simulink model "car_model_FIXED"  (R2022b)
settings: Solver=VariableStepAuto  StartTime=0.0  StopTime=60  RelTol=1e-3
values from neighbouring files (symbols this model uses):
  ABS_MAX_TORQUE = [25 25 25 25]    [Startup.m]
  ABS_MAX_TRQ_CMD = dot(ABS_MAX_TORQUE, MOTOR_ENABLE)    [Startup.m]
  ABS_MIN_TORQUE = [0.01 0.01 0.01 0.01]    [Startup.m]
  acc_IC = 0    [Startup.m]
  ACCELERATION_MAX = 30    [Startup.m]
  ang_IC = 0    [Startup.m]
  ang_vel_IC = 0    [Startup.m]
  ax = Reference_Signals.Chassis_Acceleration_VNED.ax.Data(:)    [Simulation_Data_Parse.m]    (also in Vehicle_Sim_Parse.m)
  ay = Reference_Signals.Chassis_Acceleration_VNED.ay.Data(:)    [Simulation_Data_Parse.m]    (also in Vehicle_Sim_Parse.m)
  az = Reference_Signals.Chassis_Acceleration_VNED.az.Data(:)    [Simulation_Data_Parse.m]    (also in Vehicle_Sim_Parse.m)
  battery_current_IC = 0    [Startup.m]
  BATTERY_CURRENT_MAX = 140    [Startup.m]
  BATTERY_CURRENT_MIN = 0    [Startup.m]
  battery_FT_IC = 300    [Startup.m]
  battery_T_IC = 300    [Startup.m]
  BATTERY_TEMPERATURE_MAX = 60    [Startup.m]
  BATTERY_TEMPERATURE_MIN = 0    [Startup.m]
  battery_voltage_IC = Ns*max(Em)    [Startup.m]
  BATTERY_VOLTAGE_MAX = 340    [Startup.m]
  BATTERY_VOLTAGE_MIN = 60    [Startup.m]
  Brake_Pressure_IC = 1    [Startup.m]
  ccl_IC = 0    [Startup.m]
  CENTER_STEER_ANGLE_MAX = 130    [Startup.m]
  covarience_matrix_IC = Simulink.Parameter(eye(28)./1000)    [Startup.m]
  dcl_IC = 140    [Startup.m]
  DCL_MAX = 130    [Startup.m]
  DCL_MIN = 0    [Startup.m]
  driver_t = 0.015    [Startup.m]
  fusion_t = Simulink.Parameter(0.01)    [Startup.m]
  fusion_t_sim = fusion_t.copy    [Startup.m]
  Fz_IC = m_all*g/4    [Startup.m]
  g = 9.81    [Startup.m]
  gps_hz = 0.01    [Startup.m]
  gps_ratio = Simulink.Parameter(gps_hz / imu_hz.Value)    [Startup.m]
  imu_hz = fusion_t.copy    [Startup.m]
  location_lla_IC = Simulink.Parameter([40.437675, -86.943750, 200])    [Startup.m]
  MAG_MAX = 200    [Startup.m]
  Max_Brake_Pressure = 10^8    (= 100000000)    [Startup.m]
  Max_Driver_Input = 1    [Startup.m]
  MAX_DTHETA_DRIVER = 360    [Startup.m]
  MAX_STEERING_ADJUST = 15    [Startup.m]
  Min_Brake_Pressure = 1    [Startup.m]
  Min_Driver_Input = 0    [Startup.m]
  motor_current_IC = 0    [Startup.m]
  MOTOR_CURRENT_MAX = 70    [Startup.m]
  MOTOR_CURRENT_MIN = 0    [Startup.m]
  MOTOR_ENABLE = [0 0 1 1]    [Startup.m]
  motor_FT_IC = 300    [Startup.m]
  motor_T_IC = 300    [Startup.m]
  MOTOR_TEMPERATURE_MAX = 100    [Startup.m]
  MOTOR_TEMPERATURE_MIN = 0    [Startup.m]
  motor_voltage_IC = 332    [Startup.m]
  MOTOR_VOLTAGE_MAX = 340    [Startup.m]
  MOTOR_VOLTAGE_MIN = 90    [Startup.m]
  omega_IC = 0    [Startup.m]
  OMEGA_MAX = 150    [Startup.m]
  OMEGA_MIN = 0    [Startup.m]
  ORIENTATION_MAX = 360    [Startup.m]
  pos_IC = 0    [Startup.m]
  POS_MAX = 300    [Startup.m]
  rho = 1.225    [Startup.m]
  selected_maxvm = MIN_TRACK_DATA.(event_names(10))    [Startup.m]
  selected_sweep = ALL_SWEEP_DATA.(sweep_names(1))    [Startup.m]
  selected_track = ALL_TRACK_DATA.(event_names(10))    [Startup.m]
  shock_length_IC = 0.1    [Startup.m]
  SHOCK_LENGTH_MAX = 0.25    [Startup.m]
  SHOCK_LENGTH_MIN = 0    [Startup.m]
  state_IC = zeros(28,1)    [Startup.m]
  theta_IC = 0    [Startup.m]
  TRACTION_ENABLE = 0    [Startup.m]
  TVS_ENABLE = 0    [Startup.m]
  tvs_t = 0.015    [Startup.m]
  tvs_t_sim = tvs_t    (= 0.015)    [Startup.m]
  Tx_I = 0    [Startup.m]
  vel_IC = [0 0 0]    [Startup.m]
  VELOCITY_MAX = 30    [Startup.m]
  X = Reference_Signals.Chassis_Position.X.Data(:)    [Simulation_Data_Parse.m]    (also in Vehicle_Sim_Parse.m = Chassis_Signals.InertFrm.Cg.Disp.X.Data(:))
  Y = Reference_Signals.Chassis_Position.Y.Data(:)    [Simulation_Data_Parse.m]    (also in Vehicle_Sim_Parse.m = Chassis_Signals.InertFrm.Cg.Disp.Y.Data(:))
  YAW_ENABLE = 1    [Startup.m]
  YAW_MAX = 2.5    [Startup.m]
undefined symbols (not defined in the file or in its folder): ActSuspDutyCycle, Aeq_left, Aeq_right, alpha_error, ang_acc_hystersesis, area_air, axb, br, brake_bias, covA, covG, covM, covP, covV, CURRENT_BUFFER, cy_sweep, dB, deadband_angle, dIndex, DiscIntNeverNeededParam, dt_OFF, dt_ON, dTx, dx, dZ, efficiency_grid, F0z, forward_look_straight, forward_look_turn, Fz_sweep, GAIN_ABS, gearbox_efficiency, gr, I, I_Driver, IMU_accel, IMU_gyro, IMU_mag, IMUNED2VNED, indicies, IYY, kx_sweep, l, lambda_star, low_V_SA, lr, m_all, m_body, m_unsprung, MAGNED2VNED, MAX_I_Driver, max_yaw, min_velocity_regen, motorControllerCurve, motorTempCurve, motorTempX, mu_star, mx_sweep, my_sweep, noise_state ... (+40)
libraries: fl_lib x82, nesl_utility x32, vehdynlibtire x10, vehdynlibsuspension x8, simulink x5, autolibutils x5, sharedtransform x5, sdl_lib x4, EngineCoolingComponents_lib x4, slpidlib x3, SimscapeFluids_lib x3, shared6dof x2
(part 8 of 14)

== system car_model_FIXED/Control Systems/TVS/Yaw Controller/Integrator ==
  yaw_error : Inport
  windup : Inport  Port=2
  P_control : Inport  Port=3
  control_signal : Inport  Port=4
  Constant2 : Constant  Value=0
  Gain : Gain  Gain=I*tvs_t
  Gain1 : Gain  Gain=0.5
  Sum1 : Sum  Inputs=|+-
  Sum2 : Sum  Inputs=|++
  Sum3 : Sum  Inputs=|++
  Switch1 : Switch  Criteria=u2 > Threshold  SaturateOnIntegerOverflow=off  InputSameDT=off
  Switch2 : Switch  Criteria=u2 > Threshold  SaturateOnIntegerOverflow=off  InputSameDT=off
  Unit Delay1 : UnitDelay  SampleTime=-1  HasFrameUpgradeWarning=on
  Unit Delay2 : UnitDelay  SampleTime=-1  HasFrameUpgradeWarning=on
  I_control : Outport
  wires:
  Constant2/1 -> Switch1/1
  windup/1 -> Switch1/2, Switch2/2
  Gain/1 -> Unit Delay1/1, Sum3/1
  Switch1/1 -> Sum2/1
  Gain1/1 -> Switch1/3
  Sum2/1 -> Switch2/3, I_control/1
  Unit Delay1/1 -> Sum3/2
  Sum3/1 -> Gain1/1
  yaw_error/1 -> Gain/1
  control_signal/1 -> Sum1/1
  P_control/1 -> Sum1/2
  Sum1/1 -> Switch2/1
  Switch2/1 -> Unit Delay2/1
  Unit Delay2/1 -> Sum2/2

== system car_model_FIXED/Control Systems/TVS/Yaw Controller/Windup Hysteresis ==
  max_ang_acc : Inport
  min_ang_acc : Inport  Port=2
  control_signal : Inport  Port=3
  AND : Logic  IconShape=distinctive  AllPortsSameDT=off  OutDataTypeStr=boolean
  Bias : Bias  Bias=-ang_acc_hystersesis  SaturateOnIntegerOverflow=off
  Bias1 : Bias  Bias=ang_acc_hystersesis  SaturateOnIntegerOverflow=off
  Bias2 : Bias  Bias=ang_acc_hystersesis  SaturateOnIntegerOverflow=off
  Bias3 : Bias  Bias=-ang_acc_hystersesis  SaturateOnIntegerOverflow=off
  Less Than : RelationalOperator  Operator=>  OutDataTypeStr=boolean  RndMeth=Simplest  InputSameDT=off
  Less Than1 : RelationalOperator  Operator=<  OutDataTypeStr=boolean  RndMeth=Simplest  InputSameDT=off
  Less Than2 : RelationalOperator  Operator=<  OutDataTypeStr=boolean  RndMeth=Simplest  InputSameDT=off
  Less Than3 : RelationalOperator  Operator=>  OutDataTypeStr=boolean  RndMeth=Simplest  InputSameDT=off
  NOT : Logic  Operator=NOT  IconShape=distinctive  AllPortsSameDT=off  OutDataTypeStr=boolean
  OR : Logic  Operator=OR  IconShape=distinctive  AllPortsSameDT=off  OutDataTypeStr=boolean
  Switch : Switch  Criteria=u2 > Threshold  SaturateOnIntegerOverflow=off  InputSameDT=off
  Switch1 : Switch  Criteria=u2 > Threshold  SaturateOnIntegerOverflow=off  InputSameDT=off
  Unit Delay : UnitDelay  SampleTime=-1  HasFrameUpgradeWarning=on
  windup : Outport
  wires:
  min_ang_acc/1 -> Bias1/1, Bias3/1
  max_ang_acc/1 -> Bias/1, Bias2/1
  Less Than/1 -> AND/1
  Less Than1/1 -> AND/2
  Bias/1 -> Less Than1/2
  Bias1/1 -> Less Than/2
  AND/1 -> Switch/2, NOT/1
  Unit Delay/1 -> Switch/3, windup/1  "windup"
  Bias3/1 -> Less Than2/2
  Bias2/1 -> Less Than3/2
  OR/1 -> Switch1/2, Switch1/1
  Less Than3/1 -> OR/2
  Less Than2/1 -> OR/1
  control_signal/1 -> Less Than2/1, Less Than3/1, Less Than1/1, Less Than/1
  NOT/1 -> Switch/1
  Switch/1 -> Switch1/3
  Switch1/1 -> Unit Delay/1  "windup"

== system car_model_FIXED/Driver & Environment/Longitudinal Control/ABS/ABS system ==
  lambda0 : Inport
  Vx : Inport  Port=2
  omega : Inport  Port=3
  ABS_ENABLE : Inport  Port=4
  Bias : Bias  Bias=1  SaturateOnIntegerOverflow=off
  Constant : Constant  Value=0
  Constant1 : Constant  Value=mu_star
  Divide : Product  Inputs=*/
  Equal : RelationalOperator  Operator===  OutDataTypeStr=boolean  RndMeth=Simplest  InputSameDT=off
  Gain : Gain  Gain=-1
  Gain1 : Gain  Gain=eps
  Gain2 : Gain  Gain=-g
  Gain8 : Gain  Gain=RE
  MATLAB Function : MATLAB Function  TreatAsAtomicUnit=on  SystemSampleTime=driver_t
  MATLAB Function1 : MATLAB Function  TreatAsAtomicUnit=on
  Product : Product  Inputs=1
  Product1 : Product
  Product2 : Product
  Reshape : Reshape  OutputDimensionality=Row vector (2-D)
  Reshape1 : Reshape  OutputDimensionality=Row vector (2-D)
  Sum : Sum  Inputs=|++
  Switch : Switch  Criteria=u2 ~= 0  SaturateOnIntegerOverflow=off  InputSameDT=off
  Transpose : Math  Operator=transpose
  mu : Outport
  Bx : Outport  Port=2
  OFF_FLAG : Outport  Port=3
  wires:
  omega/1 -> Reshape1/1, Product1/2  "w"
  Product2/1 -> Sum/1, Equal/1, MATLAB Function/3(v)
  MATLAB Function/1(tau) -> Bx/1  "braking torque"
  Bias/1 -> MATLAB Function/6(lambda), MATLAB Function1/1(u)  "lambda"
  Gain8/1 -> Divide/1
  lambda0/1 -> Transpose/1
  Divide/1 -> Gain/1
  Sum/1 -> Divide/2
  Equal/1 -> Gain1/1
  Constant/1 -> Equal/2
  Gain/1 -> Bias/1
  Gain1/1 -> Sum/2
  Transpose/1 -> MATLAB Function/4(lambda0)
  Reshape/1 -> MATLAB Function/1(w_fake), Gain8/1
  MATLAB Function1/1(y) -> Product/1  "mu"
  Gain2/1 -> MATLAB Function/5(vdot)
  MATLAB Function/2(d) -> OFF_FLAG/1
  Product/1 -> Switch/1, Gain2/1
  Product1/1 -> Reshape/1
  Switch/1 -> mu/1
  Constant1/1 -> Switch/3
  Vx/1 -> Product2/2
  ABS_ENABLE/1 -> Switch/2, Product2/1, Product1/1
  Reshape1/1 -> MATLAB Function/2(w)

== system car_model_FIXED/Vehicle Model/Powertrain/Motor Cooling Loop/Air Stream ==
  V : Inport
  fan command : Inport  Port=2
  Air density [kg/m^3] : Constant  Value=rho
  Constant : Constant
  Product : Product  Inputs=3
  Radiator area [m^2] : Constant  Value=area_air
  Simulink-PS Converter1 : nesl_utility/Simulink-PS Converter  PhysicalDomain=network_engine_domain  SubClassName=ps_input  LeftPortType=input  RightPortType=output  PseudoPeriodic=off  Frequencies=[]  NoiseDistribution=none  NoiseParameters=[]  Unit=kg/s  AffineConversion=off  FilteringAndDerivatives=filter  SimscapeFilterOrder=1  InputFilterTimeConstant=0.01  UdotUserProvided=0
  Sum : Sum  Inputs=|++
  Terminator : Terminator
  mdot : PMIOPort  Side=Right
  wires:
  Constant/1 -> Sum/1
  Product/1 -> Simulink-PS Converter1/1
  Radiator area [m^2]/1 -> Product/2
  Air density [kg/m^3]/1 -> Product/3
  Sum/1 -> Product/1
  fan command/1 -> Sum/2
  V/1 -> Terminator/1
  connections:
  mdot/RConn1 -- Simulink-PS Converter1/RConn1

== system car_model_FIXED/Vehicle Model/Powertrain/Motor Cooling Loop/Expansion Tank ==
  Expansion Tank : fl_lib/Thermal Liquid/Elements/Translational Mechanical Converter (TL)  mech_orientation=1  displacement_spec=foundation.enum.DisplacementSpec.Calculate  x0=0 m  interface_area=pi*0.01^2 m^2  dead_volume=pi*0.01^2 * 0.001 m^3  environment_spec=foundation.enum.pressure_spec.specified  environment_pressure=1 atm  dynamic_compressibility=0  p0=1 atm  T0=300 K
      settings: InternalSimscapePortConfiguration="{\"Bottom\":[],\"Left\":[{\"id\":\"A\",\"label\":\"A\",\"type\":\"foundation.thermal_liquid.thermal_liquid\"},{\"id\":\"C\",\"label\":\"C\",\"type\":\"foundation.mechanical.translational.translational\"},{\"id\":\"H\",\"label\":\"H\",\"type\":\"foundation.thermal.thermal\"}],\"Right\":[{\"id\":\"R\",\"label\":\"R\",\"type\":\"foundation.mechanical.translational.translational\"}],\"Top\":[]}"
  Ideal Force Source : fl_lib/Mechanical/Mechanical Sources/Ideal Force Source
  Mechanical Translational Reference : fl_lib/Mechanical/Translational Elements/Mechanical Translational Reference
  Mechanical Translational Reference1 : fl_lib/Mechanical/Translational Elements/Mechanical Translational Reference
  PS Gain : fl_lib/Physical Signals/Functions/PS Gain  gain=-1
  PS Product : fl_lib/Physical Signals/Functions/PS Product
  Perfect Insulator : fl_lib/Thermal/Thermal Elements/Perfect Insulator  T_specify=off  T_priority=None  T=0 K  T_nominal_specify=off  T_nominal_unit=K  T_nominal_value=1
  Relief Pressure (Absolute) : fl_lib/Physical Signals/Sources/PS Constant  constant=2e5
  Relief Valve : fl_lib/Thermal Liquid/Elements/Local Restriction (TL)  restriction_type=foundation.enum.restriction_type.fixed  restriction_area=pi*0.005^2 m^2  min_area=1e-10 m^2  max_area=0.005 m^2  area=pi*0.01^2 m^2  Cd=0.7  pressure_recovery=simscape.enum.onoff.on  Re_c=12
  Tank Area : fl_lib/Physical Signals/Sources/PS Constant  constant=pi*0.01^2
  Translational Hard Stop : fl_lib/Mechanical/Translational Elements/Translational Hard Stop  upper_bnd=100 m  lower_bnd=0 m  stiff_up=1e6 N/m  stiff_low=1e6 N/m  D_up=0 N/(m/s)  D_low=0 N/(m/s)  model=3  transition=0.1 mm  v_specify=off  v_priority=None  v=0 m/s  v_nominal_specify=off  v_nominal_unit=m/s  v_nominal_value=1  f_specify=off  f_priority=None  f=0 N  f_nominal_specify=off  f_nominal_unit=N  f_nominal_value=1  x_specify=on  x_priority=High  x=0 m  x_nominal_specify=off  x_nominal_unit=m  x_nominal_value=1
  P : PMIOPort  Side=Left
  connections:
  Mechanical Translational Reference/LConn1 -- Expansion Tank/LConn2
  Perfect Insulator/LConn1 -- Expansion Tank/LConn3
  Relief Valve/LConn1 -- P/RConn1
  Relief Valve/RConn1 -- Expansion Tank/LConn1
  Ideal Force Source/LConn1 -- Expansion Tank/RConn1 -- Translational Hard Stop/LConn1
  Mechanical Translational Reference1/LConn1 -- Translational Hard Stop/RConn1 -- Ideal Force Source/RConn2
  PS Gain/LConn1 -- PS Product/RConn1
  PS Gain/RConn1 -- Ideal Force Source/RConn1
  PS Product/LConn1 -- Tank Area/RConn1
  Relief Pressure (Absolute)/RConn1 -- PS Product/LConn2

== system car_model_FIXED/Vehicle Model/Powertrain/Motor Cooling Loop/Expansion Tank1 ==
  Expansion Tank : fl_lib/Thermal Liquid/Elements/Translational Mechanical Converter (TL)  mech_orientation=1  displacement_spec=foundation.enum.DisplacementSpec.Calculate  x0=0 m  interface_area=pi*0.01^2 m^2  dead_volume=pi*0.01^2 * 0.001 m^3  environment_spec=2  environment_pressure=1 atm  dynamic_compressibility=0  p0=1 atm  T0=300 K
      settings: InternalSimscapePortConfiguration="{\"Bottom\":[],\"Left\":[{\"id\":\"A\",\"label\":\"A\",\"type\":\"foundation.thermal_liquid.thermal_liquid\"},{\"id\":\"C\",\"label\":\"C\",\"type\":\"foundation.mechanical.translational.translational\"},{\"id\":\"H\",\"label\":\"H\",\"type\":\"foundation.thermal.thermal\"}],\"Right\":[{\"id\":\"R\",\"label\":\"R\",\"type\":\"foundation.mechanical.translational.translational\"}],\"Top\":[]}"
  Ideal Force Source : fl_lib/Mechanical/Mechanical Sources/Ideal Force Source
  Mechanical Translational Reference : fl_lib/Mechanical/Translational Elements/Mechanical Translational Reference
  Mechanical Translational Reference1 : fl_lib/Mechanical/Translational Elements/Mechanical Translational Reference
  PS Gain : fl_lib/Physical Signals/Functions/PS Gain  gain=-1
  PS Product : fl_lib/Physical Signals/Functions/PS Product
  Perfect Insulator : fl_lib/Thermal/Thermal Elements/Perfect Insulator  T_specify=off  T_priority=None  T=0 K  T_nominal_specify=off  T_nominal_unit=K  T_nominal_value=1
  Relief Pressure (Absolute) : fl_lib/Physical Signals/Sources/PS Constant  constant=2e5
  Relief Valve : fl_lib/Thermal Liquid/Elements/Local Restriction (TL)  restriction_type=foundation.enum.restriction_type.fixed  restriction_area=pi*0.005^2 m^2  min_area=1e-10 m^2  max_area=0.005 m^2  area=pi*0.01^2 m^2  Cd=0.7  pressure_recovery=simscape.enum.onoff.on  Re_c=12
  Tank Area : fl_lib/Physical Signals/Sources/PS Constant  constant=pi*0.01^2
  Translational Hard Stop : fl_lib/Mechanical/Translational Elements/Translational Hard Stop  upper_bnd=100 m  lower_bnd=0 m  stiff_up=1e6 N/m  stiff_low=1e6 N/m  D_up=0 N/(m/s)  D_low=0 N/(m/s)  model=3  transition=0.1 mm  v_specify=off  v_priority=None  v=0 m/s  v_nominal_specify=off  v_nominal_unit=m/s  v_nominal_value=1  f_specify=off  f_priority=None  f=0 N  f_nominal_specify=off  f_nominal_unit=N  f_nominal_value=1  x_specify=on  x_priority=High  x=0 m  x_nominal_specify=off  x_nominal_unit=m  x_nominal_value=1
  P : PMIOPort  Side=Left
  connections:
  Mechanical Translational Reference/LConn1 -- Expansion Tank/LConn2
  Perfect Insulator/LConn1 -- Expansion Tank/LConn3
  Relief Valve/LConn1 -- P/RConn1
  Relief Valve/RConn1 -- Expansion Tank/LConn1
  Ideal Force Source/LConn1 -- Expansion Tank/RConn1 -- Translational Hard Stop/LConn1
  Mechanical Translational Reference1/LConn1 -- Translational Hard Stop/RConn1 -- Ideal Force Source/RConn2
  PS Gain/LConn1 -- PS Product/RConn1
  PS Gain/RConn1 -- Ideal Force Source/RConn1
  PS Product/LConn1 -- Tank Area/RConn1
  Relief Pressure (Absolute)/RConn1 -- PS Product/LConn2

== system car_model_FIXED/Vehicle Model/Powertrain/Motor Cooling Loop/Motor FL ==
  Fluid Jacket : EngineCoolingComponents_lib/Fluid Jacket  volume=5.2e-6 m^3  length=0.087 m  area=pi*(0.012/2)^2 m^2  loss_coefficient=1  heat_transfer_area=22925 mm^2  Nu_coeff=[0.3, 0.8, 0.33]  p_I_specify=off  p_I_priority=High  p_I=1 atm  p_I_nominal_specify=off  p_I_nominal_unit=MPa  p_I_nominal_value=1  T_I_specify=on  T_I_priority=High  T_I=300 K  T_I_nominal_specify=off  T_I_nominal_unit=K  T_I_nominal_value=1
      settings: InternalSimscapePortConfiguration="{\"Bottom\":[],\"Left\":[{\"id\":\"A\",\"label\":\"A\",\"type\":\"foundation.thermal_liquid.thermal_liquid\"},{\"id\":\"H\",\"label\":\"H\",\"type\":\"foundation.thermal.thermal\"}],\"Right\":[{\"id\":\"B\",\"label\":\"B\",\"type\":\"foundation.thermal_liquid.thermal_liquid\"}],\"Top\":[]}"
  Piston Thermal Mass : fl_lib/Thermal/Thermal Elements/Thermal Mass  mass=3.1 kg  sp_heat=184.91 J/kg/K  num_ports=foundation.enum.numPorts2.one  T_specify=on  T_priority=High  T=300 K  T_nominal_specify=off  T_nominal_unit=K  T_nominal_value=1  Q_specify=off  Q_priority=None  Q=0 W  Q_nominal_specify=off  Q_nominal_unit=W  Q_nominal_value=1
  Sensor : Subsystem
      mask Display: disp('T');
  Heat In : PMIOPort  Side=Left
  Fluid In : PMIOPort  Port=2  Side=Left
  Fluid Out : PMIOPort  Port=3  Side=Right
  connections:
  Fluid Jacket/RConn1 -- Fluid Out/RConn1
  Fluid Jacket/LConn1 -- Fluid In/RConn1
  Fluid Jacket/LConn2 -- Sensor/LConn1 -- Heat In/RConn1 -- Piston Thermal Mass/LConn1

== system car_model_FIXED/Vehicle Model/Powertrain/Motor Cooling Loop/Motor FR ==
  Fluid Jacket : EngineCoolingComponents_lib/Fluid Jacket  volume=5.2e-6 m^3  length=0.087 m  area=pi*(0.012/2)^2 m^2  loss_coefficient=1  heat_transfer_area=22925 mm^2  Nu_coeff=[0.3, 0.8, 0.33]  p_I_specify=off  p_I_priority=High  p_I=1 atm  p_I_nominal_specify=off  p_I_nominal_unit=MPa  p_I_nominal_value=1  T_I_specify=on  T_I_priority=High  T_I=300 K  T_I_nominal_specify=off  T_I_nominal_unit=K  T_I_nominal_value=1
      settings: InternalSimscapePortConfiguration="{\"Bottom\":[],\"Left\":[{\"id\":\"A\",\"label\":\"A\",\"type\":\"foundation.thermal_liquid.thermal_liquid\"},{\"id\":\"H\",\"label\":\"H\",\"type\":\"foundation.thermal.thermal\"}],\"Right\":[{\"id\":\"B\",\"label\":\"B\",\"type\":\"foundation.thermal_liquid.thermal_liquid\"}],\"Top\":[]}"
  Piston Thermal Mass : fl_lib/Thermal/Thermal Elements/Thermal Mass  mass=3.1 kg  sp_heat=184.91 J/kg/K  num_ports=foundation.enum.numPorts2.one  T_specify=on  T_priority=High  T=300 K  T_nominal_specify=off  T_nominal_unit=K  T_nominal_value=1  Q_specify=off  Q_priority=None  Q=0 W  Q_nominal_specify=off  Q_nominal_unit=W  Q_nominal_value=1
  Sensor : Subsystem
      mask Display: disp('T');
  Fluid Out : PMIOPort  Side=Left
  Heat In : PMIOPort  Port=2  Side=Left
  Fluid In : PMIOPort  Port=3  Side=Right
  connections:
  Fluid Jacket/RConn1 -- Fluid Out/RConn1
  Fluid Jacket/LConn1 -- Fluid In/RConn1
  Fluid Jacket/LConn2 -- Heat In/RConn1 -- Sensor/LConn1 -- Piston Thermal Mass/LConn1

== system car_model_FIXED/Vehicle Model/Powertrain/Motor Cooling Loop/Motor RL ==
  Fluid Jacket : EngineCoolingComponents_lib/Fluid Jacket  volume=5.2e-6 m^3  length=0.087 m  area=pi*(0.012/2)^2 m^2  loss_coefficient=1  heat_transfer_area=22925 mm^2  Nu_coeff=[0.3, 0.8, 0.33]  p_I_specify=off  p_I_priority=High  p_I=1 atm  p_I_nominal_specify=off  p_I_nominal_unit=MPa  p_I_nominal_value=1  T_I_specify=on  T_I_priority=High  T_I=300 K  T_I_nominal_specify=off  T_I_nominal_unit=K  T_I_nominal_value=1
      settings: InternalSimscapePortConfiguration="{\"Bottom\":[],\"Left\":[{\"id\":\"A\",\"label\":\"A\",\"type\":\"foundation.thermal_liquid.thermal_liquid\"},{\"id\":\"H\",\"label\":\"H\",\"type\":\"foundation.thermal.thermal\"}],\"Right\":[{\"id\":\"B\",\"label\":\"B\",\"type\":\"foundation.thermal_liquid.thermal_liquid\"}],\"Top\":[]}"
  Piston Thermal Mass : fl_lib/Thermal/Thermal Elements/Thermal Mass  mass=3.1 kg  sp_heat=184.91 J/kg/K  num_ports=foundation.enum.numPorts2.one  T_specify=on  T_priority=High  T=300 K  T_nominal_specify=off  T_nominal_unit=K  T_nominal_value=1  Q_specify=off  Q_priority=None  Q=0 W  Q_nominal_specify=off  Q_nominal_unit=W  Q_nominal_value=1
  Sensor : Subsystem
      mask Display: disp('T');
  Heat In : PMIOPort  Side=Left
  Fluid In : PMIOPort  Port=2  Side=Left
  Fluid Out : PMIOPort  Port=3  Side=Right
  connections:
  Fluid Jacket/RConn1 -- Fluid Out/RConn1
  Fluid Jacket/LConn1 -- Fluid In/RConn1
  Fluid Jacket/LConn2 -- Sensor/LConn1 -- Heat In/RConn1 -- Piston Thermal Mass/LConn1

== system car_model_FIXED/Vehicle Model/Powertrain/Motor Cooling Loop/Motor RR ==
  Fluid Jacket : EngineCoolingComponents_lib/Fluid Jacket  volume=5.2e-6 m^3  length=0.087 m  area=pi*(0.012/2)^2 m^2  loss_coefficient=1  heat_transfer_area=22925 mm^2  Nu_coeff=[0.3, 0.8, 0.33]  p_I_specify=off  p_I_priority=High  p_I=1 atm  p_I_nominal_specify=off  p_I_nominal_unit=MPa  p_I_nominal_value=1  T_I_specify=on  T_I_priority=High  T_I=300 K  T_I_nominal_specify=off  T_I_nominal_unit=K  T_I_nominal_value=1
      settings: InternalSimscapePortConfiguration="{\"Bottom\":[],\"Left\":[{\"id\":\"A\",\"label\":\"A\",\"type\":\"foundation.thermal_liquid.thermal_liquid\"},{\"id\":\"H\",\"label\":\"H\",\"type\":\"foundation.thermal.thermal\"}],\"Right\":[{\"id\":\"B\",\"label\":\"B\",\"type\":\"foundation.thermal_liquid.thermal_liquid\"}],\"Top\":[]}"
  Piston Thermal Mass : fl_lib/Thermal/Thermal Elements/Thermal Mass  mass=3.1 kg  sp_heat=184.91 J/kg/K  num_ports=foundation.enum.numPorts2.one  T_specify=on  T_priority=High  T=300 K  T_nominal_specify=off  T_nominal_unit=K  T_nominal_value=1  Q_specify=off  Q_priority=None  Q=0 W  Q_nominal_specify=off  Q_nominal_unit=W  Q_nominal_value=1
  Sensor : Subsystem
      mask Display: disp('T');
  Fluid Out : PMIOPort  Side=Left
  Heat In : PMIOPort  Port=2  Side=Left
  Fluid In : PMIOPort  Port=3  Side=Right
  connections:
  Fluid Jacket/RConn1 -- Fluid Out/RConn1
  Fluid Jacket/LConn1 -- Fluid In/RConn1
  Fluid Jacket/LConn2 -- Heat In/RConn1 -- Sensor/LConn1 -- Piston Thermal Mass/LConn1

== system car_model_FIXED/Vehicle Model/Powertrain/Motor Cooling Loop/Radiator ==
  Hose : fl_lib/Thermal Liquid/Elements/Pipe (TL)  length=0.5 m  area=0.0000712557 m^2  Dh=0.009525 m  length_add=5 m  roughness=1.5e-5 m  Re_lam=2e+3  Re_tur=4e+3  shape_factor=64  Nu_lam=3.66  dynamic_compressibility=1  inertia=0  p0=1 atm  T0=300 K  mdot0=0.1 kg/s
  Hose1 : fl_lib/Thermal Liquid/Elements/Pipe (TL)  length=0.5 m  area=0.0000712557 m^2  Dh=0.009525 m  length_add=5 m  roughness=1.5e-5 m  Re_lam=2e+3  Re_tur=4e+3  shape_factor=64  Nu_lam=3.66  dynamic_compressibility=1  inertia=0  p0=1 atm  T0=300 K  mdot0=0.1 kg/s
  Perfect Insulator1 : fl_lib/Thermal/Thermal Elements/Perfect Insulator  T_specify=off  T_priority=None  T=0 K  T_nominal_specify=off  T_nominal_unit=K  T_nominal_value=1
  Perfect Insulator2 : fl_lib/Thermal/Thermal Elements/Perfect Insulator  T_specify=off  T_priority=None  T=0 K  T_nominal_specify=off  T_nominal_unit=K  T_nominal_value=1
  Radiator : SimscapeFluids_lib/Fluid Network Interfaces/Heat Exchangers/Heat Exchanger (G-TL)  hex_type=fluids.interfaces.enum.flow_arrangement_spec.cross_flow  shell_num=1  cross_type=fluids.interfaces.enum.cross_flow_heat_exchanger_G_TL_spec.unmixed_mixed  NTU_TLU=[.5, 1, 2, 3, 4, 5]  CR_TLU=[0, .25, .5, .75, 1]  eff_TLU=[.3, .3, .3, .3, .3; .6, .55, .5, .47, .43; .85, .76, .68, .61, .55; .94, .83, .72, .65, .58; .98, .86, .75, .66, .58; .99, .86, .75, .66, .58]  wall_thermal_dynamics=simscape.enum.onoff.off  thermal_mass_wall=447 J/K  R_wall=1.6e-4 K/W  min_flow_area_1=0.01 m^2  Dh_press_1=0.1 m  gas_volume_1=rad_air_vol m^3  Re_lam_1=2000  Re_tur_1=4000  pressure_loss_spec_1=fluids.interfaces.enum.pressure_loss_spec.constant  pressure_loss_coeff_1=0.1  length_press_1=1 m  length_add_1=0.1 m  roughness_1=15e-6 m  Re_friction_TLU_1=[400, 1000, 1500, 3000, 4000, 6000, 10000, 20000, 40000, 60000, 100000, 100000000]  friction_factor_TLU_1=[.264, .112, .071, .0417, .0387, .0268, .025, .0232, .0226, .022, .0214, .0214]  shape_factor_1=64  Re_Euler_TLU_1=[50, 500, 1000, 2000]  Euler_TLU_1=[4.4505, .6864, .4791, .3755]  heat_transfer_spec_1=fluids.interfaces.enum.heat_transfer_spec.constant  heat_transfer_area_1=0.4 m^2  heat_coeff_1=100 W/(m^2 * K)  length_heat_1=1 m  Nu_lam_1=3.66  Re_Colburn_TLU_1=[100, 150, 1000]  Colburn_factor_TLU_1=[.019, .013, .002]  Re_Nu_TLU_1=[100, 150, 1000]  Pr_Nu_TLU_1=[1, 10]  Nu_TLU_1=[3.72, 4.21; 3.75, 4.44; 4.21, 7.15]  fouling_factor_1=1e-4 m^2*K/W  mdot_threshold_1=1e-6 kg/s  min_heat_coeff_1=5 W/(m^2 * K)  min_flow_area_2=0.01 m^2  Dh_press_2=0.1 m  liquid_volume_2=rad_liq_vol m^3  Re_lam_2=2000  Re_tur_2=4000  pressure_loss_spec_2=fluids.interfaces.enum.pressure_loss_spec.constant  pressure_loss_coeff_2=0.1  length_press_2=1 m  length_add_2=0.1 m  roughness_2=15e-6 m  Re_friction_TLU_2=[400, 1000, 1500, 3000, 4000, 6000, 10000, 20000, 40000, 60000, 100000, 100000000]  friction_factor_TLU_2=[.264, .112, .071, .0417, .0387, .0268, .025, .0232, .0226, .022, .0214, .0214]  shape_factor_2=64  Re_Euler_TLU_2=[50, 500, 1000, 2000]  Euler_TLU_2=[4.4505, .6864, .4791, .3755]  heat_transfer_spec_2=fluids.interfaces.enum.heat_transfer_spec.constant  heat_transfer_area_2=0.4 m^2  heat_coeff_2=100 W/(m^2 * K)  length_heat_2=1 m  Nu_lam_2=3.66  Re_Colburn_TLU_2=[100, 150, 1000]  Colburn_factor_TLU_2=[.019, .013, .002]  Re_Nu_TLU_2=[100, 150, 1000]  Pr_Nu_TLU_2=[1, 10]  Nu_TLU_2=[3.72, 4.21; 3.75, 4.44; 4.21, 7.15]  fouling_factor_2=1e-4 m^2*K/W  min_heat_coeff_2=5 W/(m^2 * K)  T0_1=Tair K  p0_1=1 atm  dynamic_compressibility_2=simscape.enum.onoff.off  T0_2=motor_FT_IC K  p0_2=1 atm  mdot1_TLU=radiator.mdot_air kg/s  mdot2_TLU=radiator.mdot_liquid kg/s  SD_TLU=radiator.SD kW/K  Q_check=fluids.interfaces.enum.SD_max_check.none  mdot_dp_TLU_1=radiator.mdot_air kg/s  p_diff_TLU_1=radiator.dp_air MPa  T_ref_in_1=293.15 K  p_ref_in_1=0.101325 MPa  area_1=radiator.area_air m^2  mdot_dp_TLU_2=radiator.mdot_liquid kg/s  p_diff_TLU_2=radiator.dp_liquid MPa  T_ref_in_2=293.15 K  p_ref_in_2=0.101325 MPa  mdot_threshold_2=1e-3 kg/s  area_2=pipe.area cm^2
      settings: InternalSimscapePortConfiguration="{\"Bottom\":[],\"Left\":[{\"id\":\"A1\",\"label\":\"A1\",\"type\":\"foundation.gas.gas\"},{\"id\":\"B1\",\"label\":\"B1\",\"type\":\"foundation.gas.gas\"}],\"Right\":[{\"id\":\"A2\",\"label\":\"A2\",\"type\":\"foundation.thermal_liquid.thermal_liquid\"},{\"id\":\"B2\",\"label\":\"B2\",\"type\":\"foundation.thermal_liquid.thermal_liquid\"}],\"Top\":[]}"
  A2 : PMIOPort  Side=Left
  A1 : PMIOPort  Port=2  Side=Left
  B2 : PMIOPort  Port=3  Side=Right
  B1 : PMIOPort  Port=4  Side=Right
  connections:
  Perfect Insulator2/LConn1 -- Hose/LConn2
  Perfect Insulator1/LConn1 -- Hose1/LConn2
  Hose1/RConn1 -- Radiator/RConn1
  A2/RConn1 -- Hose1/LConn1
  Radiator/RConn2 -- Hose/LConn1
  Radiator/LConn1 -- A1/RConn1
  B1/RConn1 -- Radiator/LConn2
  B2/RConn1 -- Hose/RConn1

== system car_model_FIXED/Vehicle Model/Suspension/Double Wishbone Suspension/Steer Rate Adapter ==
  Veh : Inport
  Add : Sum
  Bus Selector3 : BusSelector  OutputSignals=BdyFrm.Cg.AngVel.r
  Constant : Constant  Value=zeros(1,4)
  Matrix Concatenate : Concatenate  NumInputs=3  Mode=Multidimensional array
  Matrix Concatenate1 : Concatenate  NumInputs=3  Mode=Multidimensional array
  Reshape2 : Reshape  OutputDimensionality=Row vector (2-D)
  Reshape3 : Reshape  OutputDimensionality=Row vector (2-D)
  Reshape4 : Reshape  OutputDimensionality=Row vector (2-D)
  Selector3 : Selector  InputPortWidth=1  IndexOptions=Index vector (dialog)  Indices=[1 1 1 1]  OutputSizes=1
  SteerRates : Constant  Value=zeros(1,4)
  AngVel : Outport  VectorParamsAs1DForOutWhenUnconnected=off
  wires:
  Reshape2/1 -> Matrix Concatenate1/1, Matrix Concatenate1/3, Matrix Concatenate1/2
  Constant/1 -> Reshape3/1
  Selector3/1 -> Reshape4/1
  Bus Selector3/1 -> Selector3/1  "<r>"
  Matrix Concatenate/1 -> Add/2
  SteerRates/1 -> Reshape2/1
  Reshape4/1 -> Matrix Concatenate/3
  Reshape3/1 -> Matrix Concatenate/2, Matrix Concatenate/1
  Matrix Concatenate1/1 -> Add/1
  Veh/1 -> Bus Selector3/1
  Add/1 -> AngVel/1  "AngVel"

== system car_model_FIXED/Vehicle Model/Suspension/Double Wishbone Suspension/Steering Adapter ==
  Steer : Inport
  Reshape1 : Reshape  OutputDimensionality=Row vector (2-D)
  Selector : Selector  IndexOptions=Index vector (dialog)  Indices=[1 2]  OutputSizes=1
  Steering Model : Subsystem
  StrgAng : Outport  VectorParamsAs1DForOutWhenUnconnected=off
  wires:
  Reshape1/1 -> StrgAng/1
  Selector/1 -> Reshape1/1
  Steering Model/1(steering_angles) -> Selector/1
  Steer/1 -> Steering Model/1(steering_angle)

== system car_model_FIXED/Vehicle Model/Suspension/Double Wishbone Suspension/Vehicle Adapter ==
  Veh : Inport
  Bus Creator3 : BusCreator  Inputs=2
  Bus Selector1 : BusSelector  OutputSignals=InertFrm.FrntAxl.Lft.Disp.X,InertFrm.FrntAxl.Lft.Disp.Y,InertFrm.FrntAxl.Lft.Disp.Z,InertFrm.FrntAxl.Rght.Disp.X,InertFrm.FrntAxl.Rght.Disp.Y,InertFrm.FrntAxl.Rght.Disp.Z,InertFrm.RearAxl.Lft.Disp.X,InertFrm.RearAxl.Lft.Disp.Y,InertFrm.RearAxl.Lft.Disp.Z,InertFrm.RearAxl.Rght.Disp.X,InertFrm.RearAxl.Rght.Disp.Y,InertFrm.RearAxl.Rght.Disp.Z
  Bus Selector2 : BusSelector  OutputSignals=BdyFrm.FrntAxl.Lft.Vel.xdot,BdyFrm.FrntAxl.Lft.Vel.ydot,BdyFrm.FrntAxl.Lft.Vel.zdot,BdyFrm.FrntAxl.Rght.Vel.xdot,BdyFrm.FrntAxl.Rght.Vel.ydot,BdyFrm.FrntAxl.Rght.Vel.zdot,BdyFrm.RearAxl.Lft.Vel.xdot,BdyFrm.RearAxl.Lft.Vel.ydot,BdyFrm.RearAxl.Lft.Vel.zdot,BdyFrm.RearAxl.Rght.Vel.xdot,BdyFrm.RearAxl.Rght.Vel.ydot,BdyFrm.RearAxl.Rght.Vel.zdot
  Bus Selector3 : BusSelector  OutputSignals=InertFrm.FrntAxl.Lft.Vel.Xdot,InertFrm.FrntAxl.Lft.Vel.Ydot,InertFrm.FrntAxl.Lft.Vel.Zdot,InertFrm.FrntAxl.Rght.Vel.Xdot,InertFrm.FrntAxl.Rght.Vel.Ydot,InertFrm.FrntAxl.Rght.Vel.Zdot,InertFrm.RearAxl.Lft.Vel.Xdot,InertFrm.RearAxl.Lft.Vel.Ydot,InertFrm.RearAxl.Lft.Vel.Zdot,InertFrm.RearAxl.Rght.Vel.Xdot,InertFrm.RearAxl.Rght.Vel.Ydot,InertFrm.RearAxl.Rght.Vel.Zdot
  Inertial Frame CG to Axle Offset : Constant  Value=[zeros(2,4);dZ*ones(1,4)]
  Mux1 : Mux  Inputs=12
  Mux2 : Mux  Inputs=12
  Mux3 : Mux  Inputs=12
  Reshape : Reshape  OutputDimensionality=Customize  OutputDimensions=[3,4]
  Reshape1 : Reshape  OutputDimensionality=Customize  OutputDimensions=[3,4]
  Reshape2 : Reshape  OutputDimensionality=Customize  OutputDimensions=[3,4]
  Sum : Sum  Inputs=|+-
  VehSusp : Outport  VectorParamsAs1DForOutWhenUnconnected=off
  VehVbody : Outport  Port=2  VectorParamsAs1DForOutWhenUnconnected=off
  wires:
  Veh/1 -> Bus Selector3/1, Bus Selector2/1, Bus Selector1/1
  Reshape2/1 -> VehVbody/1  "V"
  Bus Creator3/1 -> VehSusp/1  "Veh"
  Reshape/1 -> Sum/1
  Bus Selector1/1 -> Mux2/1  "<X>"
  Bus Selector1/2 -> Mux2/2  "<Y>"
  Bus Selector1/3 -> Mux2/3  "<Z>"
  Bus Selector1/4 -> Mux2/4  "<X>"
  Bus Selector1/5 -> Mux2/5  "<Y>"
  Bus Selector1/6 -> Mux2/6  "<Z>"
  Bus Selector1/7 -> Mux2/7  "<X>"
  Bus Selector1/8 -> Mux2/8  "<Y>"
  Bus Selector1/9 -> Mux2/9  "<Z>"
  Bus Selector1/10 -> Mux2/10  "<X>"
  Bus Selector1/11 -> Mux2/11  "<Y>"
  Bus Selector1/12 -> Mux2/12  "<Z>"
  Bus Selector2/1 -> Mux1/1  "<xdot>"
  Bus Selector2/2 -> Mux1/2  "<ydot>"
  Bus Selector2/3 -> Mux1/3  "<zdot>"
  Bus Selector2/4 -> Mux1/4  "<xdot>"
  Bus Selector2/5 -> Mux1/5  "<ydot>"
  Bus Selector2/6 -> Mux1/6  "<zdot>"
  Bus Selector2/7 -> Mux1/7  "<xdot>"
  Bus Selector2/8 -> Mux1/8  "<ydot>"
  Bus Selector2/9 -> Mux1/9  "<zdot>"
  Bus Selector2/10 -> Mux1/10  "<xdot>"
  Bus Selector2/11 -> Mux1/11  "<ydot>"
  Bus Selector2/12 -> Mux1/12  "<zdot>"
  Mux1/1 -> Reshape2/1
  Mux2/1 -> Reshape/1
  Inertial Frame CG to Axle Offset/1 -> Sum/2
  Sum/1 -> Bus Creator3/1  "P"
  Mux3/1 -> Reshape1/1
  Bus Selector3/12 -> Mux3/12  "<Zdot>"
  Bus Selector3/11 -> Mux3/11  "<Ydot>"
  Bus Selector3/10 -> Mux3/10  "<Xdot>"
  Bus Selector3/9 -> Mux3/9  "<Zdot>"
  Bus Selector3/8 -> Mux3/8  "<Ydot>"
  Bus Selector3/7 -> Mux3/7  "<Xdot>"
  Bus Selector3/6 -> Mux3/6  "<Zdot>"
  Bus Selector3/5 -> Mux3/5  "<Ydot>"
  Bus Selector3/4 -> Mux3/4  "<Xdot>"
  Bus Selector3/3 -> Mux3/3  "<Zdot>"
  Bus Selector3/2 -> Mux3/2  "<Ydot>"
  Bus Selector3/1 -> Mux3/1  "<Xdot>"
  Reshape1/1 -> Bus Creator3/2  "V"

== system car_model_FIXED/Vehicle Model/Suspension/Double Wishbone Suspension/Wheel  Adapter ==
  Wheels : Inport
  Bus Selector : BusSelector  OutputSignals=SuspFrame.Fx,SuspFrame.Fy
  Bus Selector1 : BusSelector  OutputSignals=SuspFrame.Re
  Bus Selector2 : BusSelector  OutputSignals=SuspFrame.Mx,SuspFrame.My,SuspFrame.Mz
  Bus Selector3 : BusSelector  OutputSignals=SuspFrame.z,SuspFrame.zdot
  Matrix Concatenate : Concatenate  NumInputs=3  Mode=Multidimensional array
  Reshape{,1..7} (8 alike) : Reshape  OutputDimensionality=Row vector (2-D)
  WhlFx : Outport  VectorParamsAs1DForOutWhenUnconnected=off
  WhlFy : Outport  Port=2  VectorParamsAs1DForOutWhenUnconnected=off
  z : Outport  Port=3  VectorParamsAs1DForOutWhenUnconnected=off
  zdot : Outport  Port=4  VectorParamsAs1DForOutWhenUnconnected=off
  M : Outport  Port=5  VectorParamsAs1DForOutWhenUnconnected=off
  Re : Outport  Port=6  VectorParamsAs1DForOutWhenUnconnected=off
  wires:
  Reshape7/1 -> WhlFy/1
  Reshape6/1 -> WhlFx/1
  Bus Selector/1 -> Reshape6/1  "<Fx>"
  Bus Selector/2 -> Reshape7/1  "<Fy>"
  Bus Selector3/1 -> Reshape/1  "<z>"
  Wheels/1 -> Bus Selector1/1, Bus Selector2/1, Bus Selector3/1, Bus Selector/1
  Bus Selector3/2 -> Reshape2/1  "<zdot>"
  Reshape2/1 -> zdot/1  "zdot"
  Bus Selector1/1 -> Reshape1/1  "<Re>"
  Reshape1/1 -> Re/1  "Re"
  Bus Selector2/1 -> Reshape3/1  "<Mx>"
  Bus Selector2/2 -> Reshape4/1  "<My>"
  Bus Selector2/3 -> Reshape5/1  "<Mz>"
  Reshape3/1 -> Matrix Concatenate/1
  Reshape4/1 -> Matrix Concatenate/2
  Reshape5/1 -> Matrix Concatenate/3
  Matrix Concatenate/1 -> M/1  "M"
  Reshape/1 -> z/1  "z"

== system car_model_FIXED/Vehicle Model/Suspension/Independent Mapped Front Suspension Mapped Solid Axle Rear Suspension/Steer Rate Adapter ==
  Veh : Inport
  Add : Sum
  Bus Selector3 : BusSelector  OutputSignals=BdyFrm.Cg.AngVel.r
  Constant : Constant  Value=zeros(1,4)
  Matrix Concatenate : Concatenate  NumInputs=3  Mode=Multidimensional array
  Matrix Concatenate1 : Concatenate  NumInputs=3  Mode=Multidimensional array
  Reshape2 : Reshape  OutputDimensionality=Row vector (2-D)
  Reshape3 : Reshape  OutputDimensionality=Row vector (2-D)
  Reshape4 : Reshape  OutputDimensionality=Row vector (2-D)
  Selector3 : Selector  InputPortWidth=1  IndexOptions=Index vector (dialog)  Indices=[1 1 1 1]  OutputSizes=1
  SteerRates : Constant  Value=zeros(1,4)
  AngVel : Outport  VectorParamsAs1DForOutWhenUnconnected=off
  wires:
  Reshape2/1 -> Matrix Concatenate1/1, Matrix Concatenate1/3, Matrix Concatenate1/2
  Constant/1 -> Reshape3/1
  Selector3/1 -> Reshape4/1
  Bus Selector3/1 -> Selector3/1  "<r>"
  Matrix Concatenate/1 -> Add/2
  SteerRates/1 -> Reshape2/1
  Reshape4/1 -> Matrix Concatenate/3
  Reshape3/1 -> Matrix Concatenate/2, Matrix Concatenate/1
  Matrix Concatenate1/1 -> Add/1
  Veh/1 -> Bus Selector3/1
  Add/1 -> AngVel/1  "AngVel"

== system car_model_FIXED/Vehicle Model/Suspension/Independent Mapped Front Suspension Mapped Solid Axle Rear Suspension/Steering Adapter ==
  Steer : Inport
  Reshape1 : Reshape  OutputDimensionality=Row vector (2-D)
  Selector : Selector  IndexOptions=Index vector (dialog)  Indices=[1 2]  OutputSizes=1
  StrgAng : Outport  VectorParamsAs1DForOutWhenUnconnected=off
  wires:
  Reshape1/1 -> StrgAng/1
  Steer/1 -> Selector/1
  Selector/1 -> Reshape1/1

== system car_model_FIXED/Vehicle Model/Suspension/Independent Mapped Front Suspension Mapped Solid Axle Rear Suspension/Vehicle Adapter ==
  Veh : Inport
  Bus Creator3 : BusCreator  Inputs=2
  Bus Selector1 : BusSelector  OutputSignals=InertFrm.FrntAxl.Lft.Disp.X,InertFrm.FrntAxl.Lft.Disp.Y,InertFrm.FrntAxl.Lft.Disp.Z,InertFrm.FrntAxl.Rght.Disp.X,InertFrm.FrntAxl.Rght.Disp.Y,InertFrm.FrntAxl.Rght.Disp.Z,InertFrm.RearAxl.Lft.Disp.X,InertFrm.RearAxl.Lft.Disp.Y,InertFrm.RearAxl.Lft.Disp.Z,InertFrm.RearAxl.Rght.Disp.X,InertFrm.RearAxl.Rght.Disp.Y,InertFrm.RearAxl.Rght.Disp.Z
  Bus Selector2 : BusSelector  OutputSignals=BdyFrm.FrntAxl.Lft.Vel.xdot,BdyFrm.FrntAxl.Lft.Vel.ydot,BdyFrm.FrntAxl.Lft.Vel.zdot,BdyFrm.FrntAxl.Rght.Vel.xdot,BdyFrm.FrntAxl.Rght.Vel.ydot,BdyFrm.FrntAxl.Rght.Vel.zdot,BdyFrm.RearAxl.Lft.Vel.xdot,BdyFrm.RearAxl.Lft.Vel.ydot,BdyFrm.RearAxl.Lft.Vel.zdot,BdyFrm.RearAxl.Rght.Vel.xdot,BdyFrm.RearAxl.Rght.Vel.ydot,BdyFrm.RearAxl.Rght.Vel.zdot
  Bus Selector3 : BusSelector  OutputSignals=InertFrm.FrntAxl.Lft.Vel.Xdot,InertFrm.FrntAxl.Lft.Vel.Ydot,InertFrm.FrntAxl.Lft.Vel.Zdot,InertFrm.FrntAxl.Rght.Vel.Xdot,InertFrm.FrntAxl.Rght.Vel.Ydot,InertFrm.FrntAxl.Rght.Vel.Zdot,InertFrm.RearAxl.Lft.Vel.Xdot,InertFrm.RearAxl.Lft.Vel.Ydot,InertFrm.RearAxl.Lft.Vel.Zdot,InertFrm.RearAxl.Rght.Vel.Xdot,InertFrm.RearAxl.Rght.Vel.Ydot,InertFrm.RearAxl.Rght.Vel.Zdot
  Inertial Frame CG to Axle Offset : Constant  Value=[zeros(2,4);VEH.HeightCG*ones(1,4)]
  Mux1 : Mux  Inputs=12
  Mux2 : Mux  Inputs=12
  Mux3 : Mux  Inputs=12
  Reshape : Reshape  OutputDimensionality=Customize  OutputDimensions=[3,4]
  Reshape1 : Reshape  OutputDimensionality=Customize  OutputDimensions=[3,4]
  Reshape2 : Reshape  OutputDimensionality=Customize  OutputDimensions=[3,4]
  Sum : Sum  Inputs=|+-
  VehSusp : Outport  VectorParamsAs1DForOutWhenUnconnected=off
  VehVbody : Outport  Port=2  VectorParamsAs1DForOutWhenUnconnected=off
  wires:
  Veh/1 -> Bus Selector3/1, Bus Selector2/1, Bus Selector1/1
  Reshape2/1 -> VehVbody/1  "V"
  Bus Creator3/1 -> VehSusp/1  "Veh"
  Reshape/1 -> Sum/1
  Bus Selector1/1 -> Mux2/1  "<X>"
  Bus Selector1/2 -> Mux2/2  "<Y>"
  Bus Selector1/3 -> Mux2/3  "<Z>"
  Bus Selector1/4 -> Mux2/4  "<X>"
  Bus Selector1/5 -> Mux2/5  "<Y>"
  Bus Selector1/6 -> Mux2/6  "<Z>"
  Bus Selector1/7 -> Mux2/7  "<X>"
  Bus Selector1/8 -> Mux2/8  "<Y>"
  Bus Selector1/9 -> Mux2/9  "<Z>"
  Bus Selector1/10 -> Mux2/10  "<X>"
  Bus Selector1/11 -> Mux2/11  "<Y>"
  Bus Selector1/12 -> Mux2/12  "<Z>"
  Bus Selector2/1 -> Mux1/1  "<xdot>"
  Bus Selector2/2 -> Mux1/2  "<ydot>"
  Bus Selector2/3 -> Mux1/3  "<zdot>"
  Bus Selector2/4 -> Mux1/4  "<xdot>"
  Bus Selector2/5 -> Mux1/5  "<ydot>"
  Bus Selector2/6 -> Mux1/6  "<zdot>"
  Bus Selector2/7 -> Mux1/7  "<xdot>"
  Bus Selector2/8 -> Mux1/8  "<ydot>"
  Bus Selector2/9 -> Mux1/9  "<zdot>"
  Bus Selector2/10 -> Mux1/10  "<xdot>"
  Bus Selector2/11 -> Mux1/11  "<ydot>"
  Bus Selector2/12 -> Mux1/12  "<zdot>"
  Mux1/1 -> Reshape2/1
  Mux2/1 -> Reshape/1
  Inertial Frame CG to Axle Offset/1 -> Sum/2
  Sum/1 -> Bus Creator3/1  "P"
  Mux3/1 -> Reshape1/1
  Bus Selector3/12 -> Mux3/12  "<Zdot>"
  Bus Selector3/11 -> Mux3/11  "<Ydot>"
  Bus Selector3/10 -> Mux3/10  "<Xdot>"
  Bus Selector3/9 -> Mux3/9  "<Zdot>"
  Bus Selector3/8 -> Mux3/8  "<Ydot>"
  Bus Selector3/7 -> Mux3/7  "<Xdot>"
  Bus Selector3/6 -> Mux3/6  "<Zdot>"
  Bus Selector3/5 -> Mux3/5  "<Ydot>"
  Bus Selector3/4 -> Mux3/4  "<Xdot>"
  Bus Selector3/3 -> Mux3/3  "<Zdot>"
  Bus Selector3/2 -> Mux3/2  "<Ydot>"
  Bus Selector3/1 -> Mux3/1  "<Xdot>"
  Reshape1/1 -> Bus Creator3/2  "V"

== system car_model_FIXED/Vehicle Model/Suspension/Independent Mapped Front Suspension Mapped Solid Axle Rear Suspension/Wheel  Adapter ==
  Wheels : Inport
  Bus Selector : BusSelector  OutputSignals=SuspFrame.Fx,SuspFrame.Fy
  Bus Selector1 : BusSelector  OutputSignals=SuspFrame.Re
  Bus Selector2 : BusSelector  OutputSignals=SuspFrame.Mx,SuspFrame.My,SuspFrame.Mz
  Bus Selector3 : BusSelector  OutputSignals=SuspFrame.z,SuspFrame.zdot
  Matrix Concatenate : Concatenate  NumInputs=3  Mode=Multidimensional array
  Reshape{,1..7} (8 alike) : Reshape  OutputDimensionality=Row vector (2-D)
  WhlFx : Outport  VectorParamsAs1DForOutWhenUnconnected=off
  WhlFy : Outport  Port=2  VectorParamsAs1DForOutWhenUnconnected=off
  z : Outport  Port=3  VectorParamsAs1DForOutWhenUnconnected=off
  zdot : Outport  Port=4  VectorParamsAs1DForOutWhenUnconnected=off
  M : Outport  Port=5  VectorParamsAs1DForOutWhenUnconnected=off
  Re : Outport  Port=6  VectorParamsAs1DForOutWhenUnconnected=off
  wires:
  Reshape7/1 -> WhlFy/1
  Reshape6/1 -> WhlFx/1
  Bus Selector/1 -> Reshape6/1  "<Fx>"
  Bus Selector/2 -> Reshape7/1  "<Fy>"
  Bus Selector3/1 -> Reshape/1  "<z>"
  Wheels/1 -> Bus Selector1/1, Bus Selector2/1, Bus Selector3/1, Bus Selector/1
  Bus Selector3/2 -> Reshape2/1  "<zdot>"
  Reshape2/1 -> zdot/1  "zdot"
  Bus Selector1/1 -> Reshape1/1  "<Re>"
  Reshape1/1 -> Re/1  "Re"
  Bus Selector2/1 -> Reshape3/1  "<Mx>"
  Bus Selector2/2 -> Reshape4/1  "<My>"
  Bus Selector2/3 -> Reshape5/1  "<Mz>"
  Reshape3/1 -> Matrix Concatenate/1
  Reshape4/1 -> Matrix Concatenate/2
  Reshape5/1 -> Matrix Concatenate/3
  Matrix Concatenate/1 -> M/1  "M"
  Reshape/1 -> z/1  "z"

== system car_model_FIXED/Vehicle Model/Suspension/Kinematics and Compliance Independent Suspension/Calculate dynamic track width from lateral wheel center displacement change ==
  dWhlY : Inport
  dWhlZ : Inport  Port=2
  Front Track Calculation : Subsystem
  Gain : Gain  Gain=-1
  Rear Track Calculation : Subsystem
  Sign : Signum  ZeroCross=off
  Vector Concatenate : Concatenate
  w : Outport
  wires:
  dWhlZ/1 -> Gain/1
  dWhlY/1 -> Rear Track Calculation/1(dWhlY), Front Track Calculation/1(dWhlY)
  Vector Concatenate/1 -> w/1
  Front Track Calculation/1(w_front) -> Vector Concatenate/1
  Rear Track Calculation/1(w_rear) -> Vector Concatenate/2
  Sign/1 -> Rear Track Calculation/2(sign), Front Track Calculation/2(sign)
  Gain/1 -> Sign/1

== system car_model_FIXED/Vehicle Model/Suspension/Kinematics and Compliance Independent Suspension/Steer Rate Adapter ==
  Veh : Inport
  Add : Sum
  Bus Selector3 : BusSelector  OutputSignals=BdyFrm.Cg.AngVel.r
  Constant : Constant  Value=zeros(1,4)
  Matrix Concatenate : Concatenate  NumInputs=3  Mode=Multidimensional array
  Matrix Concatenate1 : Concatenate  NumInputs=3  Mode=Multidimensional array
  Reshape2 : Reshape  OutputDimensionality=Row vector (2-D)
  Reshape3 : Reshape  OutputDimensionality=Row vector (2-D)
  Reshape4 : Reshape  OutputDimensionality=Row vector (2-D)
  Selector3 : Selector  InputPortWidth=1  IndexOptions=Index vector (dialog)  Indices=[1 1 1 1]  OutputSizes=1
  SteerRates : Constant  Value=zeros(1,4)
  AngVel : Outport  VectorParamsAs1DForOutWhenUnconnected=off
  wires:
  Reshape2/1 -> Matrix Concatenate1/1, Matrix Concatenate1/3, Matrix Concatenate1/2
  Constant/1 -> Reshape3/1
  Selector3/1 -> Reshape4/1
  Bus Selector3/1 -> Selector3/1  "<r>"
  Matrix Concatenate/1 -> Add/2
  SteerRates/1 -> Reshape2/1
  Reshape4/1 -> Matrix Concatenate/3
  Reshape3/1 -> Matrix Concatenate/2, Matrix Concatenate/1
  Matrix Concatenate1/1 -> Add/1
  Veh/1 -> Bus Selector3/1
  Add/1 -> AngVel/1  "AngVel"

== system car_model_FIXED/Vehicle Model/Suspension/Kinematics and Compliance Independent Suspension/Steering Adapter ==
  Steer : Inport
  Reshape1 : Reshape  OutputDimensionality=Row vector (2-D)
  Selector : Selector  IndexOptions=Index vector (dialog)  Indices=[1 2]  OutputSizes=1
  StrgAng : Outport  VectorParamsAs1DForOutWhenUnconnected=off
  wires:
  Reshape1/1 -> StrgAng/1
  Steer/1 -> Selector/1
  Selector/1 -> Reshape1/1

== system car_model_FIXED/Vehicle Model/Suspension/Kinematics and Compliance Independent Suspension/Vehicle Adapter ==
  Veh : Inport
  Bus Creator3 : BusCreator  Inputs=2
  Bus Selector1 : BusSelector  OutputSignals=InertFrm.FrntAxl.Lft.Disp.X,InertFrm.FrntAxl.Lft.Disp.Y,InertFrm.FrntAxl.Lft.Disp.Z,InertFrm.FrntAxl.Rght.Disp.X,InertFrm.FrntAxl.Rght.Disp.Y,InertFrm.FrntAxl.Rght.Disp.Z,InertFrm.RearAxl.Lft.Disp.X,InertFrm.RearAxl.Lft.Disp.Y,InertFrm.RearAxl.Lft.Disp.Z,InertFrm.RearAxl.Rght.Disp.X,InertFrm.RearAxl.Rght.Disp.Y,InertFrm.RearAxl.Rght.Disp.Z
  Bus Selector2 : BusSelector  OutputSignals=BdyFrm.FrntAxl.Lft.Vel.xdot,BdyFrm.FrntAxl.Lft.Vel.ydot,BdyFrm.FrntAxl.Lft.Vel.zdot,BdyFrm.FrntAxl.Rght.Vel.xdot,BdyFrm.FrntAxl.Rght.Vel.ydot,BdyFrm.FrntAxl.Rght.Vel.zdot,BdyFrm.RearAxl.Lft.Vel.xdot,BdyFrm.RearAxl.Lft.Vel.ydot,BdyFrm.RearAxl.Lft.Vel.zdot,BdyFrm.RearAxl.Rght.Vel.xdot,BdyFrm.RearAxl.Rght.Vel.ydot,BdyFrm.RearAxl.Rght.Vel.zdot
  Bus Selector3 : BusSelector  OutputSignals=InertFrm.FrntAxl.Lft.Vel.Xdot,InertFrm.FrntAxl.Lft.Vel.Ydot,InertFrm.FrntAxl.Lft.Vel.Zdot,InertFrm.FrntAxl.Rght.Vel.Xdot,InertFrm.FrntAxl.Rght.Vel.Ydot,InertFrm.FrntAxl.Rght.Vel.Zdot,InertFrm.RearAxl.Lft.Vel.Xdot,InertFrm.RearAxl.Lft.Vel.Ydot,InertFrm.RearAxl.Lft.Vel.Zdot,InertFrm.RearAxl.Rght.Vel.Xdot,InertFrm.RearAxl.Rght.Vel.Ydot,InertFrm.RearAxl.Rght.Vel.Zdot
  Inertial Frame CG to Axle Offset : Constant  Value=[zeros(2,4);VEH.HeightCG*ones(1,4)]
  Mux1 : Mux  Inputs=12
  Mux2 : Mux  Inputs=12
  Mux3 : Mux  Inputs=12
  Reshape : Reshape  OutputDimensionality=Customize  OutputDimensions=[3,4]
  Reshape1 : Reshape  OutputDimensionality=Customize  OutputDimensions=[3,4]
  Reshape2 : Reshape  OutputDimensionality=Customize  OutputDimensions=[3,4]
  Sum : Sum  Inputs=|+-
  VehSusp : Outport  VectorParamsAs1DForOutWhenUnconnected=off
  VehVbody : Outport  Port=2  VectorParamsAs1DForOutWhenUnconnected=off
  wires:
  Veh/1 -> Bus Selector3/1, Bus Selector2/1, Bus Selector1/1
  Reshape2/1 -> VehVbody/1  "V"
  Bus Creator3/1 -> VehSusp/1  "Veh"
  Reshape/1 -> Sum/1
  Bus Selector1/1 -> Mux2/1  "<X>"
  Bus Selector1/2 -> Mux2/2  "<Y>"
  Bus Selector1/3 -> Mux2/3  "<Z>"
  Bus Selector1/4 -> Mux2/4  "<X>"
  Bus Selector1/5 -> Mux2/5  "<Y>"
  Bus Selector1/6 -> Mux2/6  "<Z>"
  Bus Selector1/7 -> Mux2/7  "<X>"
  Bus Selector1/8 -> Mux2/8  "<Y>"
  Bus Selector1/9 -> Mux2/9  "<Z>"
  Bus Selector1/10 -> Mux2/10  "<X>"
  Bus Selector1/11 -> Mux2/11  "<Y>"
  Bus Selector1/12 -> Mux2/12  "<Z>"
  Bus Selector2/1 -> Mux1/1  "<xdot>"
  Bus Selector2/2 -> Mux1/2  "<ydot>"
  Bus Selector2/3 -> Mux1/3  "<zdot>"
  Bus Selector2/4 -> Mux1/4  "<xdot>"
  Bus Selector2/5 -> Mux1/5  "<ydot>"
  Bus Selector2/6 -> Mux1/6  "<zdot>"
  Bus Selector2/7 -> Mux1/7  "<xdot>"
  Bus Selector2/8 -> Mux1/8  "<ydot>"
  Bus Selector2/9 -> Mux1/9  "<zdot>"
  Bus Selector2/10 -> Mux1/10  "<xdot>"
  Bus Selector2/11 -> Mux1/11  "<ydot>"
  Bus Selector2/12 -> Mux1/12  "<zdot>"
  Mux1/1 -> Reshape2/1
  Mux2/1 -> Reshape/1
  Inertial Frame CG to Axle Offset/1 -> Sum/2
  Sum/1 -> Bus Creator3/1  "P"
  Mux3/1 -> Reshape1/1
  Bus Selector3/12 -> Mux3/12  "<Zdot>"
  Bus Selector3/11 -> Mux3/11  "<Ydot>"
  Bus Selector3/10 -> Mux3/10  "<Xdot>"
  Bus Selector3/9 -> Mux3/9  "<Zdot>"
  Bus Selector3/8 -> Mux3/8  "<Ydot>"
  Bus Selector3/7 -> Mux3/7  "<Xdot>"
  Bus Selector3/6 -> Mux3/6  "<Zdot>"
  Bus Selector3/5 -> Mux3/5  "<Ydot>"
  Bus Selector3/4 -> Mux3/4  "<Xdot>"
  Bus Selector3/3 -> Mux3/3  "<Zdot>"
  Bus Selector3/2 -> Mux3/2  "<Ydot>"
  Bus Selector3/1 -> Mux3/1  "<Xdot>"
  Reshape1/1 -> Bus Creator3/2  "V"

== system car_model_FIXED/Vehicle Model/Suspension/Kinematics and Compliance Independent Suspension/Wheel  Adapter ==
  Wheels : Inport
  Bus Selector : BusSelector  OutputSignals=SuspFrame.Fx,SuspFrame.Fy
  Bus Selector1 : BusSelector  OutputSignals=SuspFrame.Re
  Bus Selector2 : BusSelector  OutputSignals=SuspFrame.Mx,SuspFrame.My,SuspFrame.Mz
  Bus Selector3 : BusSelector  OutputSignals=SuspFrame.z,SuspFrame.zdot
  Matrix Concatenate : Concatenate  NumInputs=3  Mode=Multidimensional array
  Reshape{,1..7} (8 alike) : Reshape  OutputDimensionality=Row vector (2-D)
  WhlFx : Outport  VectorParamsAs1DForOutWhenUnconnected=off
  WhlFy : Outport  Port=2  VectorParamsAs1DForOutWhenUnconnected=off
  z : Outport  Port=3  VectorParamsAs1DForOutWhenUnconnected=off
  zdot : Outport  Port=4  VectorParamsAs1DForOutWhenUnconnected=off
  M : Outport  Port=5  VectorParamsAs1DForOutWhenUnconnected=off
  Re : Outport  Port=6  VectorParamsAs1DForOutWhenUnconnected=off
  wires:
  Reshape7/1 -> WhlFy/1
  Reshape6/1 -> WhlFx/1
  Bus Selector/1 -> Reshape6/1  "<Fx>"
  Bus Selector/2 -> Reshape7/1  "<Fy>"
  Bus Selector3/1 -> Reshape/1  "<z>"
  Wheels/1 -> Bus Selector1/1, Bus Selector2/1, Bus Selector3/1, Bus Selector/1
  Bus Selector3/2 -> Reshape2/1  "<zdot>"
  Reshape2/1 -> zdot/1  "zdot"
  Bus Selector1/1 -> Reshape1/1  "<Re>"
  Reshape1/1 -> Re/1  "Re"
  Bus Selector2/1 -> Reshape3/1  "<Mx>"
  Bus Selector2/2 -> Reshape4/1  "<My>"
  Bus Selector2/3 -> Reshape5/1  "<Mz>"
  Reshape3/1 -> Matrix Concatenate/1
  Reshape4/1 -> Matrix Concatenate/2
  Reshape5/1 -> Matrix Concatenate/3
  Matrix Concatenate/1 -> M/1  "M"
  Reshape/1 -> z/1  "z"
